simulink model "CoupledWaterTank"  (R2018a)
settings: Solver=VariableStepAuto  StartTime=0.0  StopTime=300  RelTol=1e-3
undefined symbols (not defined in the file or in its folder): Advantech, PCI
libraries: sldrtlib x2
settings Model: Creator=lvandeke  LastModifiedBy=lvandeke

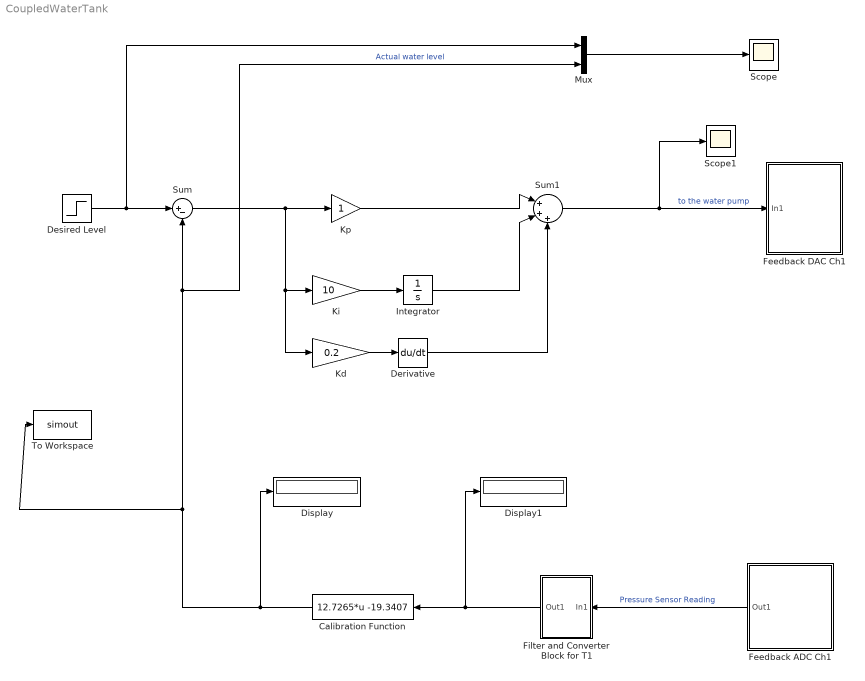
== system CoupledWaterTank ==
  Calibration Function : Fcn  Expr=12.7265*u -19.3407
  Derivative : Derivative
  Desired Level : Step  Time=0  After=7  SampleTime=0
  Display : Display
  Display1 : Display
  Feedback ADC Ch1 : Subsystem  mask{Tsamp=0.1}
      mask prompts: Tsamp "Sampling time"
      mask Display:
      | image(imread('bckg.bmp'))
      | disp('PCI1711 \n Lab I/O Board \n\n Feedback  ADC')
  Feedback DAC Ch1 : Subsystem  mask(DAC Unit for Feedback Experiments){st=0.1, ch=1}
      mask prompts: st "Sample Time"; ch "Output Channel"
      mask help:
      | Digital to Analog Output  for Feedback Experiments
      | using Advantech PCI1711  I/O board
      mask Display:
      | image(imread('bckg.bmp'))
      | disp('PCI1711 \n Lab I/O Board \n\n Feedback  DAC')
  Filter and Converter Block for T1 : Subsystem
      mask Display:
      | image(imread('bckg.bmp'))
      | disp('Filter \n & \n Converter')
  Integrator : Integrator
  Kd : Gain  Gain=0.2
  Ki : Gain  Gain=10
  Kp : Gain
  Mux : Mux  Inputs=2
  Scope : Scope
  Scope1 : Scope
  Sum : Sum  Inputs=|+-
  Sum1 : Sum  Inputs=|+++
  To Workspace : ToWorkspace  VariableName=simout  SaveFormat=Timeseries  SampleTime=-1
  wires:
  Mux/1 -> Scope/1
  Kd/1 -> Derivative/1
  Derivative/1 -> Sum1/3
  Filter and Converter Block for T1/1(Out1) -> Display1/1, Calibration Function/1
  Sum/1 -> Kd/1, Ki/1, Kp/1
  Desired Level/1 -> Mux/1, Sum/1
  Sum1/1 -> Scope1/1, Feedback DAC Ch1/1(In1)  "to the water pump"
  Ki/1 -> Integrator/1
  Calibration Function/1 -> To Workspace/1, Mux/2, Sum/2, Display/1  "Actual water level"
  Feedback ADC Ch1/1(Out1) -> Filter and Converter Block for T1/1(In1)  "Pressure Sensor Reading"
  Integrator/1 -> Sum1/2
  Kp/1 -> Sum1/1

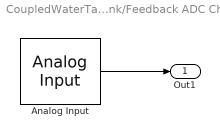
== system CoupledWaterTank/Feedback ADC Ch1 ==
  Analog Input : sldrtlib/Analog Input  SampleTime=Tsamp  MaxMissedTicks=10  ShowMissedTicks=off  YieldWhenWaiting=off  DrvName=Advantech/PCI-1711  DrvAddress=4294967295  DrvOptions=zeros(1,0)  Channels=2  RangeMode=1  VoltRange=1  DataType=1
      settings: AttributesFormatString=Advantech\nPCI-1711 [auto]  SourceProductName=Simulink Desktop Real-Time
  Out1 : Outport
  wires:
  Analog Input/1 -> Out1/1

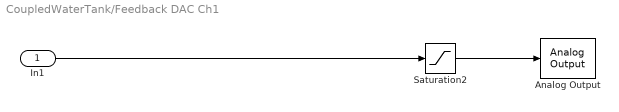
== system CoupledWaterTank/Feedback DAC Ch1 ==
  In1 : Inport
  Analog Output : sldrtlib/Analog Output  SampleTime=st  MaxMissedTicks=10  ShowMissedTicks=off  YieldWhenWaiting=off  DrvName=Advantech/PCI-1711  DrvAddress=4294967295  DrvOptions=zeros(1,0)  Channels=ch  RangeMode=1  VoltRange=2  InitialValue=0  FinalValue=0
      settings: AttributesFormatString=Advantech\nPCI-1711 [auto]  SourceProductName=Simulink Desktop Real-Time
  Saturation2 : Saturate  UpperLimit=5  LowerLimit=0
  wires:
  In1/1 -> Saturation2/1
  Saturation2/1 -> Analog Output/1

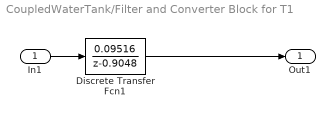
== system CoupledWaterTank/Filter and Converter Block for T1 ==
  In1 : Inport
  Discrete Transfer Fcn1 : DiscreteTransferFcn  Numerator=[0.09516]  Denominator=[1 -0.9048]  SampleTime=0.1
  Out1 : Outport
  wires:
  In1/1 -> Discrete Transfer Fcn1/1
  Discrete Transfer Fcn1/1 -> Out1/1
